simulink library "amg_clcd_lib"  (R2015b)
settings: Solver=ode3  SolverMode=SingleTasking  StartTime=0.0  StopTime=10.0  RelTol=1e-3
(part 1 of 3)
settings Model: Creator=Krisada  LastModifiedBy=Aimagin
settings DataIOCC: SaveFormat=Array  SignalLoggingSaveFormat=ModelDataLogs
settings OptimizationCC: ExpressionDepthLimit=2147483647  OptimizeModelRefInitCode=on  LifeSpan=1
settings DebuggingCC: UnderspecifiedInitializationDetection=Classic  MergeDetectMultiDrivingBlocksExec=none  SolverPrmCheckMsg=warning  FcnCallInpInsideContextMsg=UseLocalSettings  StateNameClashWarn=warning  StrictBusMsg=Warning
settings HardwareCC: ProdBitPerPointer=32  ProdLargestAtomicFloat=None  ProdIntDivRoundTo=Undefined  ProdWordSize=32  ProdHWDeviceType=ARM Compatible->Cortex - M4  TargetEndianess=LittleEndian  TargetHWDeviceType=ARM Compatible->Cortex - M4
settings RTWCC: SystemTargetFile=stm32f4.tlc  GenerateMakefile=off  TemplateMakefile=ert_default_tmf  Description=STM32F4 Target
settings CodeAppCC: IgnoreCustomStorageClasses=off  CustomSymbolStrType=$N$R$M  InternalIdentifier=Classic
settings STFCustomTargetCC: ModelReferenceCompliant=off  ConcurrentExecutionCompliant=off  GeneratePreprocessorConditionals=Use local settings  CombineOutputUpdateFcns=on  ERTCustomFileBanners=on  SupportContinuousTime=off  SupportNonInlinedSFcns=off  MATLABClassNameForMDSCustomization=Simulink.SoftwareTarget.ERTCustomization  CPPClassGenCompliant=off  GRTInterface=off  SystemTargetFile=stm32f4.tlc
settings ERTTargetCC: ModelReferenceCompliant=off  ParMdlRefBuildCompliant=off  CompOptLevelCompliant=off  ConcurrentExecutionCompliant=off  ERTFirstTimeCompliant=off  ModelStepFunctionPrototypeControlCompliant=off  CPPClassGenCompliant=off  UseToolchainInfoCompliant=off  ERTSrcFileBannerTemplate=stm32f4_code_template.cgt  ERTHdrFileBannerTemplate=stm32f4_code_template.cgt  ERTDataSrcFileTemplate=stm32f4_code_template.cgt  ERTDataHdrFileTemplate=stm32f4_code_template.cgt  ERTCustomFileTemplate=stm32f4_file_process.tlc
settings ConfigComp: CovModelRefEnable=Off

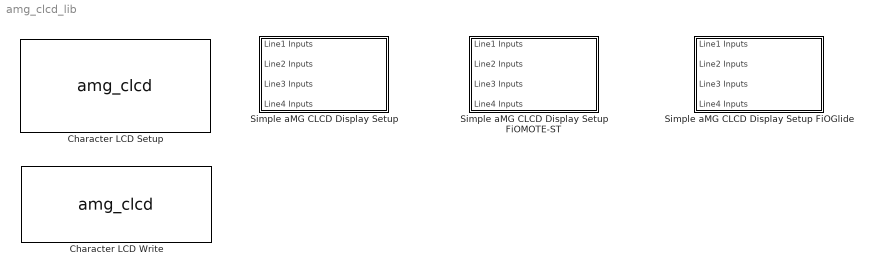
== system amg_clcd_lib ==
  Character LCD Setup : S-Function  FunctionName=amg_clcd  Parameters=module,configuration,inputtypearray,outputtypearray,confstr,sampletime,sampletimestr,blockid  SFunctionDeploymentMode=off  EnableBusSupport=off  mask(amg_clcd){configuration=Setup, module=1, model=amg CLCD Std, interface=4-bits, linecount=4, columncount=16, gpiotype=Push-pull, controlport=E, control_rs=7, control_rw=8, control_en=9, dataport_low=C, dataport=E, datalow0=8, datalow1=9, datalow2=10, datalow3=11, data0=12, data1=13, data2=14, data3=15, usestringbuffer=off, stringbuffer=<empty>, varname=, inputtypearray=[0], outputtypearray=[0], confstr=["4","4","16","PP","E","7","9","8","C","E","8","9","10","11","12","13","14","15","0","","0","0","1","0","1","0","0","0","0","stm32f0"], sampletime=-1, sampletimestr=0, blockid=CharacterLCDSetup}
      mask prompts: model "LCD model:"; linecount "Number of lines (2 or 4):"; columncount "Number of columns (16 or 20):"; gpiotype "GPIO Output type:"; controlport "GPIO control port:"; control_rs "GPIO control pin, RS:"; control_rw "GPIO control pin, RW:"; control_en "GPIO control pin, EN:"; dataport_low "GPIO data D[3:0] port"; dataport "GPIO data D[7:4] port"; datalow0 "GPIO data pin, D0:"; datalow1 "GPIO data pin, D1:"; datalow2 "GPIO data pin, D2:"; datalow3 "GPIO data pin, D3:"; data0 "GPIO data pin, D4:"; data1 "GPIO data pin, D5:"; data2 "GPIO data pin, D6:"; data3 "GPIO data pin, D7:"; usestringbuffer "Use string buffer"; stringbuffer "String buffer"; varname "Variable name"; inputtypearray "Input type array"; outputtypearray "Output type array"; confstr "Configuration string"; sampletime "Sample time (sec)"; sampletimestr "Compiled sample time (sec) in string"
      mask help:
      | Interface:
      |  - Select LCD data pin count to 4 or 8 line.
      |
      | Number of columns:
      |  - Select 16 for LCD 1x16, 2x16 or 4x16 characters.
      |  - Select 20 for LCD 1x20, 2x20 or 4x20 characters.
      |
      | GPIO Output type:
      |  - Select Push-Pull to drive 3.3V push-pull from MCU.
      |  - Select Open-Drain to allow external 5V pull-up.
      mask init:
      | amg_clcd_callback('init');
      mask Help: web(fullfile(waijungdocroot,'amg_clcd_setup.htm'), '-browser')
      mask TypeOptions configuration: Setup | Transaction
      mask Callback configuration: amg_clcd_callback('configuration');
      mask TypeOptions module: 1 | 2 | 3 | 4
      mask TypeOptions model: amg CLCD Std
      mask TypeOptions interface: 4-bits | 8-bits
      mask Callback interface: amg_clcd_callback('interface');
      mask TypeOptions gpiotype: Push-pull | Open-drain
      mask TypeOptions controlport: A | B | C | D | E | F | G | H | I
      mask TypeOptions control_rs: 0 | 1 | 2 | 3 | 4 | 5 | 6 | 7 | 8 | 9 | 10 | 11 | 12 | 13 | 14 | 15
      mask TypeOptions control_rw: 0 | 1 | 2 | 3 | 4 | 5 | 6 | 7 | 8 | 9 | 10 | 11 | 12 | 13 | 14 | 15
      mask TypeOptions control_en: 0 | 1 | 2 | 3 | 4 | 5 | 6 | 7 | 8 | 9 | 10 | 11 | 12 | 13 | 14 | 15
      mask TypeOptions dataport_low: A | B | C | D | E | F | G | H | I
      mask TypeOptions dataport: A | B | C | D | E | F | G | H | I
      mask TypeOptions datalow0: 0 | 1 | 2 | 3 | 4 | 5 | 6 | 7 | 8 | 9 | 10 | 11 | 12 | 13 | 14 | 15
      mask TypeOptions datalow1: 0 | 1 | 2 | 3 | 4 | 5 | 6 | 7 | 8 | 9 | 10 | 11 | 12 | 13 | 14 | 15
      mask TypeOptions datalow2: 0 | 1 | 2 | 3 | 4 | 5 | 6 | 7 | 8 | 9 | 10 | 11 | 12 | 13 | 14 | 15
      mask TypeOptions datalow3: 0 | 1 | 2 | 3 | 4 | 5 | 6 | 7 | 8 | 9 | 10 | 11 | 12 | 13 | 14 | 15
      mask TypeOptions data0: 0 | 1 | 2 | 3 | 4 | 5 | 6 | 7 | 8 | 9 | 10 | 11 | 12 | 13 | 14 | 15
      mask TypeOptions data1: 0 | 1 | 2 | 3 | 4 | 5 | 6 | 7 | 8 | 9 | 10 | 11 | 12 | 13 | 14 | 15
      mask TypeOptions data2: 0 | 1 | 2 | 3 | 4 | 5 | 6 | 7 | 8 | 9 | 10 | 11 | 12 | 13 | 14 | 15
      mask TypeOptions data3: 0 | 1 | 2 | 3 | 4 | 5 | 6 | 7 | 8 | 9 | 10 | 11 | 12 | 13 | 14 | 15
      mask Callback usestringbuffer: amg_clcd_callback('usestringbuffer');
      mask TypeOptions stringbuffer: <empty>
      mask Callback varname: amg_clcd_callback('varname');
      mask Callback confstr: amg_clcd_callback('confstr');
      mask Callback sampletime: amg_clcd_callback('sampletime');
      mask Callback sampletimestr: amg_clcd_callback('sampletimestr');
      mask Callback blockid: amg_clcd_callback('blockid');
      mask Display: text(0.5, 0.5, 'Module: CLCD1 (Setup)\nInterface: 4-bits\nCntrl: E7/E8/E9\nD[7:4]: E12/E13/E14/E15\nTs (sec): 0','ver','middle','hor','center');
  Character LCD Write : S-Function  FunctionName=amg_clcd  Parameters=module,configuration,inputtypearray,outputtypearray,confstr,sampletime,sampletimestr,blockid  SFunctionDeploymentMode=off  EnableBusSupport=off  mask(amg_clcd){configuration=Transaction, module=1, model=amg CLCD Std, interface=4-bits, linecount=4, columncount=20, gpiotype=Push-pull, controlport=E, control_rs=15, control_rw=13, control_en=11, dataport=A, data0=7, data1=5, data2=3, data3=1, usestringbuffer=off, stringbuffer=<empty>, varname=, inputtypearray=[4 -1 -1 -1 -1], outputtypearray=[0], confstr=["4","4","20","PP","E","15","11","13","","A","","","","","7","5","3","1","0","","1","0","0","0","1","0","0","0","0","stm32f0"], sampletime=-1, sampletimestr=0, blockid=CharacterLCDWrite}
      mask prompts: model "LCD model:"; linecount "Number of lines:"; columncount "Number of columns:"; gpiotype "GPIO Output type:"; controlport "GPIO control port:"; control_rs "GPIO control pin, RS:"; control_rw "GPIO control pin, RW:"; control_en "GPIO control pin, EN:"; dataport "GPIO data D[7:4] port"; data0 "GPIO data pin, D4:"; data1 "GPIO data pin, D5:"; data2 "GPIO data pin, D6:"; data3 "GPIO data pin, D7:"; usestringbuffer "Use string buffer"; stringbuffer "String buffer"; varname "Variable name"; inputtypearray "Input type array"; outputtypearray "Output type array"; confstr "Configuration string"; sampletime "Sample time (sec)"; sampletimestr "Compiled sample time (sec) in string"
      mask help:
      | Note for cmd:
      | 1 - Clear specified LCD line display before write data to LCD.
      | Otherwise (e.g. 0) - Write data without clearing LCD Line.
      |
      | Position:
      | x = 0, First Character (from left to right)
      | y = 0, Top Line
      mask init:
      | amg_clcd_callback('init');
      mask Help: web(fullfile(waijungdocroot,'amg_clcd_write.htm'), '-browser')
      mask TypeOptions configuration: Setup | Transaction
      mask Callback configuration: amg_clcd_callback('configuration');
      mask TypeOptions module: 1 | 2 | 3 | 4
      mask TypeOptions model: amg CLCD Std
      mask TypeOptions interface: 4-bits
      mask TypeOptions gpiotype: Push-pull | Open-drain
      mask TypeOptions controlport: A | B | C | D | E | F | G | H | I
      mask TypeOptions control_rs: 0 | 1 | 2 | 3 | 4 | 5 | 6 | 7 | 8 | 9 | 10 | 11 | 12 | 13 | 14 | 15
      mask TypeOptions control_rw: 0 | 1 | 2 | 3 | 4 | 5 | 6 | 7 | 8 | 9 | 10 | 11 | 12 | 13 | 14 | 15
      mask TypeOptions control_en: 0 | 1 | 2 | 3 | 4 | 5 | 6 | 7 | 8 | 9 | 10 | 11 | 12 | 13 | 14 | 15
      mask TypeOptions dataport: A | B | C | D | E | F | G | H | I
      mask TypeOptions data0: 0 | 1 | 2 | 3 | 4 | 5 | 6 | 7 | 8 | 9 | 10 | 11 | 12 | 13 | 14 | 15
      mask TypeOptions data1: 0 | 1 | 2 | 3 | 4 | 5 | 6 | 7 | 8 | 9 | 10 | 11 | 12 | 13 | 14 | 15
      mask TypeOptions data2: 0 | 1 | 2 | 3 | 4 | 5 | 6 | 7 | 8 | 9 | 10 | 11 | 12 | 13 | 14 | 15
      mask TypeOptions data3: 0 | 1 | 2 | 3 | 4 | 5 | 6 | 7 | 8 | 9 | 10 | 11 | 12 | 13 | 14 | 15
      mask Callback usestringbuffer: amg_clcd_callback('usestringbuffer');
      mask TypeOptions stringbuffer: Line1 | Line2 | Line3 | Line4 | Line1 | Line2 | Line3 | Line4 | Line1 | Line2 | Line3 | Line4 | <empty>
      mask Callback varname: amg_clcd_callback('varname');
      mask Callback confstr: amg_clcd_callback('confstr');
      mask Callback sampletime: amg_clcd_callback('sampletime');
      mask Callback sampletimestr: amg_clcd_callback('sampletimestr');
      mask Callback blockid: amg_clcd_callback('blockid');
      mask Display: text(0.5, 0.5, 'Module: CLCD1 (Write)\nTs (sec): 0','ver','middle','hor','center');port_label('input', 1,'cmd');port_label('input', 2,'xpos');port_label('input', 3,'ypos');port_label('input', 4,'str');
  Simple aMG CLCD Display Setup : Subsystem
      settings: CopyFcn=set_param(gcbh, 'LinkStatus', 'none')
  Simple aMG CLCD Display Setup FiOGlide : Subsystem
      settings: CopyFcn=set_param(gcbh, 'LinkStatus', 'none')
  Simple aMG CLCD Display Setup FiOMOTE-ST : Subsystem
      settings: CopyFcn=set_param(gcbh, 'LinkStatus', 'none')

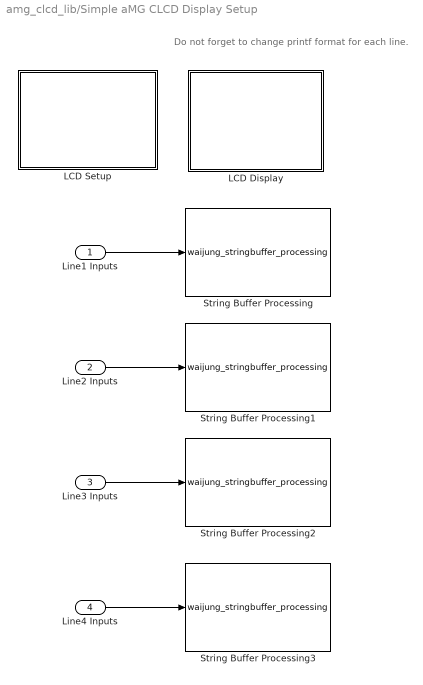
== system amg_clcd_lib/Simple aMG CLCD Display Setup ==
  note: Do not forget to change printf format for each line.
  Line1 Inputs : Inport
  Line2 Inputs : Inport  Port=2
  Line3 Inputs : Inport  Port=3
  Line4 Inputs : Inport  Port=4
  LCD Display : Subsystem
  LCD Setup : Subsystem
  String Buffer Processing : S-Function  FunctionName=waijung_stringbuffer_processing  Parameters=configuration,varname,sformat,porttypes,portcount,inputtypearray,outputtypearray,sampletime,sampletimestr,blockid  SFunctionDeploymentMode=off  EnableBusSupport=off  mask(waijung_stringbuffer_processing){configuration=sprintf, storagename=Line1, sformat='%u', enableoutput=off, varname=SimpleaMGCLCDDisplaySetupLCDSetupVolatileDataStorage_Line1, inputtypearray=[1 -1], outputtypearray=[0], porttypes=["uint32_t"], portcount=1, sampletime=-1, sampletimestr=0, blockid=SimpleaMGCLCDDisplaySetupStringBufferProcessing}
      mask prompts: configuration "Function"; storagename "String buffer"; sformat "Printf format"; enableoutput "Enable output status"; varname "Variable name"; inputtypearray "Input type array"; outputtypearray "Output type array"; porttypes "Port type list"; portcount "Port type count"; sampletime "Sample time (sec)"; sampletimestr "Compiled sample time (sec) in string"
      mask help:
      | This block implements string processing, sprintf/ sscanf command.
      | Supported format:
      | %u, %i, %o, %x: uint32
      | %d: int32
      | %e, %g, %f: single
      | %c: int8
      |
      | Status:
      |  0: Failed.
      |  Non-zero: Success.
      mask init:
      | waijung_stringbuffer_processing_callback('init');
      mask Help: web(fullfile(waijungdocroot,'String_Buffer_Processing.htm'))
      mask TypeOptions configuration: sprintf | sscanf
      mask Callback configuration: waijung_stringbuffer_processing_callback('configuration');
      mask TypeOptions storagename: Line1 | Line2 | Line3 | Line4 | Line1 | Line2 | Line3 | Line4 | Line1 | Line2 | Line3 | Line4 | <output>
      mask Callback sformat: waijung_stringbuffer_processing_callback('sformat');
      mask Callback enableoutput: waijung_stringbuffer_processing_callback('enableoutput');
      mask Callback sampletime: waijung_stringbuffer_processing_callback('sampletime');
      mask Callback sampletimestr: waijung_stringbuffer_processing_callback('sampletimestr');
      mask Callback blockid: waijung_stringbuffer_processing_callback('blockid');
      mask Display: text(0.5, 0.5, '[ sprintf ]\nBuffer: Line1\nTs (sec): 0','ver','middle','hor','center');port_label('input', 1,'%u');
  String Buffer Processing1 : S-Function  FunctionName=waijung_stringbuffer_processing  Parameters=configuration,varname,sformat,porttypes,portcount,inputtypearray,outputtypearray,sampletime,sampletimestr,blockid  SFunctionDeploymentMode=off  EnableBusSupport=off  mask(waijung_stringbuffer_processing){configuration=sprintf, storagename=Line2, sformat='%u', enableoutput=off, varname=SimpleaMGCLCDDisplaySetupLCDSetupVolatileDataStorage1_Line2, inputtypearray=[1 -1], outputtypearray=[0], porttypes=["uint32_t"], portcount=1, sampletime=-1, sampletimestr=0, blockid=SimpleaMGCLCDDisplaySetupStringBufferProcessing1}
      mask prompts: configuration "Function"; storagename "String buffer"; sformat "Printf format"; enableoutput "Enable output status"; varname "Variable name"; inputtypearray "Input type array"; outputtypearray "Output type array"; porttypes "Port type list"; portcount "Port type count"; sampletime "Sample time (sec)"; sampletimestr "Compiled sample time (sec) in string"
      mask help:
      | This block implements string processing, sprintf/ sscanf command.
      | Supported format:
      | %u, %i, %o, %x: uint32
      | %d: int32
      | %e, %g, %f: single
      | %c: int8
      |
      | Status:
      |  0: Failed.
      |  Non-zero: Success.
      mask init:
      | waijung_stringbuffer_processing_callback('init');
      mask Help: web(fullfile(waijungdocroot,'String_Buffer_Processing.htm'))
      mask TypeOptions configuration: sprintf | sscanf
      mask Callback configuration: waijung_stringbuffer_processing_callback('configuration');
      mask TypeOptions storagename: Line1 | Line2 | Line3 | Line4 | Line1 | Line2 | Line3 | Line4 | Line1 | Line2 | Line3 | Line4 | <output>
      mask Callback sformat: waijung_stringbuffer_processing_callback('sformat');
      mask Callback enableoutput: waijung_stringbuffer_processing_callback('enableoutput');
      mask Callback sampletime: waijung_stringbuffer_processing_callback('sampletime');
      mask Callback sampletimestr: waijung_stringbuffer_processing_callback('sampletimestr');
      mask Callback blockid: waijung_stringbuffer_processing_callback('blockid');
      mask Display: text(0.5, 0.5, '[ sprintf ]\nBuffer: Line2\nTs (sec): 0','ver','middle','hor','center');port_label('input', 1,'%u');
  String Buffer Processing2 : S-Function  FunctionName=waijung_stringbuffer_processing  Parameters=configuration,varname,sformat,porttypes,portcount,inputtypearray,outputtypearray,sampletime,sampletimestr,blockid  SFunctionDeploymentMode=off  EnableBusSupport=off  mask(waijung_stringbuffer_processing){configuration=sprintf, storagename=Line3, sformat='%u', enableoutput=off, varname=SimpleaMGCLCDDisplaySetupLCDSetupVolatileDataStorage2_Line3, inputtypearray=[1 -1], outputtypearray=[0], porttypes=["uint32_t"], portcount=1, sampletime=-1, sampletimestr=0, blockid=SimpleaMGCLCDDisplaySetupStringBufferProcessing2}
      mask prompts: configuration "Function"; storagename "String buffer"; sformat "Printf format"; enableoutput "Enable output status"; varname "Variable name"; inputtypearray "Input type array"; outputtypearray "Output type array"; porttypes "Port type list"; portcount "Port type count"; sampletime "Sample time (sec)"; sampletimestr "Compiled sample time (sec) in string"
      mask help:
      | This block implements string processing, sprintf/ sscanf command.
      | Supported format:
      | %u, %i, %o, %x: uint32
      | %d: int32
      | %e, %g, %f: single
      | %c: int8
      |
      | Status:
      |  0: Failed.
      |  Non-zero: Success.
      mask init:
      | waijung_stringbuffer_processing_callback('init');
      mask Help: web(fullfile(waijungdocroot,'String_Buffer_Processing.htm'))
      mask TypeOptions configuration: sprintf | sscanf
      mask Callback configuration: waijung_stringbuffer_processing_callback('configuration');
      mask TypeOptions storagename: Line1 | Line2 | Line3 | Line4 | Line1 | Line2 | Line3 | Line4 | Line1 | Line2 | Line3 | Line4 | <output>
      mask Callback sformat: waijung_stringbuffer_processing_callback('sformat');
      mask Callback enableoutput: waijung_stringbuffer_processing_callback('enableoutput');
      mask Callback sampletime: waijung_stringbuffer_processing_callback('sampletime');
      mask Callback sampletimestr: waijung_stringbuffer_processing_callback('sampletimestr');
      mask Callback blockid: waijung_stringbuffer_processing_callback('blockid');
      mask Display: text(0.5, 0.5, '[ sprintf ]\nBuffer: Line3\nTs (sec): 0','ver','middle','hor','center');port_label('input', 1,'%u');
  String Buffer Processing3 : S-Function  FunctionName=waijung_stringbuffer_processing  Parameters=configuration,varname,sformat,porttypes,portcount,inputtypearray,outputtypearray,sampletime,sampletimestr,blockid  SFunctionDeploymentMode=off  EnableBusSupport=off  mask(waijung_stringbuffer_processing){configuration=sprintf, storagename=Line4, sformat='%u', enableoutput=off, varname=SimpleaMGCLCDDisplaySetupLCDSetupVolatileDataStorage3_Line4, inputtypearray=[1 -1], outputtypearray=[0], porttypes=["uint32_t"], portcount=1, sampletime=-1, sampletimestr=0, blockid=SimpleaMGCLCDDisplaySetupStringBufferProcessing3}
      mask prompts: configuration "Function"; storagename "String buffer"; sformat "Printf format"; enableoutput "Enable output status"; varname "Variable name"; inputtypearray "Input type array"; outputtypearray "Output type array"; porttypes "Port type list"; portcount "Port type count"; sampletime "Sample time (sec)"; sampletimestr "Compiled sample time (sec) in string"
      mask help:
      | This block implements string processing, sprintf/ sscanf command.
      | Supported format:
      | %u, %i, %o, %x: uint32
      | %d: int32
      | %e, %g, %f: single
      | %c: int8
      |
      | Status:
      |  0: Failed.
      |  Non-zero: Success.
      mask init:
      | waijung_stringbuffer_processing_callback('init');
      mask Help: web(fullfile(waijungdocroot,'String_Buffer_Processing.htm'))
      mask TypeOptions configuration: sprintf | sscanf
      mask Callback configuration: waijung_stringbuffer_processing_callback('configuration');
      mask TypeOptions storagename: Line1 | Line2 | Line3 | Line4 | Line1 | Line2 | Line3 | Line4 | Line1 | Line2 | Line3 | Line4 | <output>
      mask Callback sformat: waijung_stringbuffer_processing_callback('sformat');
      mask Callback enableoutput: waijung_stringbuffer_processing_callback('enableoutput');
      mask Callback sampletime: waijung_stringbuffer_processing_callback('sampletime');
      mask Callback sampletimestr: waijung_stringbuffer_processing_callback('sampletimestr');
      mask Callback blockid: waijung_stringbuffer_processing_callback('blockid');
      mask Display: text(0.5, 0.5, '[ sprintf ]\nBuffer: Line4\nTs (sec): 0','ver','middle','hor','center');port_label('input', 1,'%u');
  wires:
  Line1 Inputs/1 -> String Buffer Processing/1
  Line2 Inputs/1 -> String Buffer Processing1/1
  Line3 Inputs/1 -> String Buffer Processing2/1
  Line4 Inputs/1 -> String Buffer Processing3/1

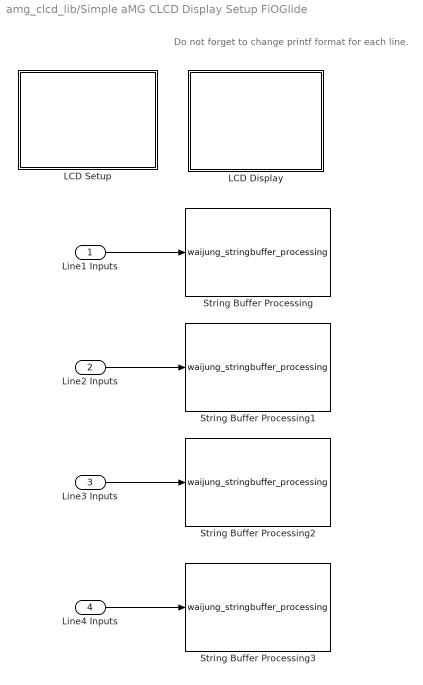
== system amg_clcd_lib/Simple aMG CLCD Display Setup FiOGlide ==
  note: Do not forget to change printf format for each line.
  Line1 Inputs : Inport
  Line2 Inputs : Inport  Port=2
  Line3 Inputs : Inport  Port=3
  Line4 Inputs : Inport  Port=4
  LCD Display : Subsystem
  LCD Setup : Subsystem
  String Buffer Processing : S-Function  FunctionName=waijung_stringbuffer_processing  Parameters=configuration,varname,sformat,porttypes,portcount,inputtypearray,outputtypearray,sampletime,sampletimestr,blockid  SFunctionDeploymentMode=off  EnableBusSupport=off  mask(waijung_stringbuffer_processing){configuration=sprintf, storagename=Line1, sformat='%u', enableoutput=off, varname=SimpleaMGCLCDDisplaySetupLCDSetupVolatileDataStorage_Line1, inputtypearray=[1 -1], outputtypearray=[0], porttypes=["uint32_t"], portcount=1, sampletime=-1, sampletimestr=0, blockid=SimpleaMGCLCDDisplaySetupStringBufferProcessing}
      mask prompts: configuration "Function"; storagename "String buffer"; sformat "Printf format"; enableoutput "Enable output status"; varname "Variable name"; inputtypearray "Input type array"; outputtypearray "Output type array"; porttypes "Port type list"; portcount "Port type count"; sampletime "Sample time (sec)"; sampletimestr "Compiled sample time (sec) in string"
      mask help:
      | This block implements string processing, sprintf/ sscanf command.
      | Supported format:
      | %u, %i, %o, %x: uint32
      | %d: int32
      | %e, %g, %f: single
      | %c: int8
      |
      | Status:
      |  0: Failed.
      |  Non-zero: Success.
      mask init:
      | waijung_stringbuffer_processing_callback('init');
      mask Help: web(fullfile(waijungdocroot,'String_Buffer_Processing.htm'))
      mask TypeOptions configuration: sprintf | sscanf
      mask Callback configuration: waijung_stringbuffer_processing_callback('configuration');
      mask TypeOptions storagename: Line1 | Line2 | Line3 | Line4 | Line1 | Line2 | Line3 | Line4 | Line1 | Line2 | Line3 | Line4 | <output>
      mask Callback sformat: waijung_stringbuffer_processing_callback('sformat');
      mask Callback enableoutput: waijung_stringbuffer_processing_callback('enableoutput');
      mask Callback sampletime: waijung_stringbuffer_processing_callback('sampletime');
      mask Callback sampletimestr: waijung_stringbuffer_processing_callback('sampletimestr');
      mask Callback blockid: waijung_stringbuffer_processing_callback('blockid');
      mask Display: text(0.5, 0.5, '[ sprintf ]\nBuffer: Line1\nTs (sec): 0','ver','middle','hor','center');port_label('input', 1,'%u');
  String Buffer Processing1 : S-Function  FunctionName=waijung_stringbuffer_processing  Parameters=configuration,varname,sformat,porttypes,portcount,inputtypearray,outputtypearray,sampletime,sampletimestr,blockid  SFunctionDeploymentMode=off  EnableBusSupport=off  mask(waijung_stringbuffer_processing){configuration=sprintf, storagename=Line2, sformat='%u', enableoutput=off, varname=SimpleaMGCLCDDisplaySetupLCDSetupVolatileDataStorage1_Line2, inputtypearray=[1 -1], outputtypearray=[0], porttypes=["uint32_t"], portcount=1, sampletime=-1, sampletimestr=0, blockid=SimpleaMGCLCDDisplaySetupStringBufferProcessing1}
      mask prompts: configuration "Function"; storagename "String buffer"; sformat "Printf format"; enableoutput "Enable output status"; varname "Variable name"; inputtypearray "Input type array"; outputtypearray "Output type array"; porttypes "Port type list"; portcount "Port type count"; sampletime "Sample time (sec)"; sampletimestr "Compiled sample time (sec) in string"
      mask help:
      | This block implements string processing, sprintf/ sscanf command.
      | Supported format:
      | %u, %i, %o, %x: uint32
      | %d: int32
      | %e, %g, %f: single
      | %c: int8
      |
      | Status:
      |  0: Failed.
      |  Non-zero: Success.
      mask init:
      | waijung_stringbuffer_processing_callback('init');
      mask Help: web(fullfile(waijungdocroot,'String_Buffer_Processing.htm'))
      mask TypeOptions configuration: sprintf | sscanf
      mask Callback configuration: waijung_stringbuffer_processing_callback('configuration');
      mask TypeOptions storagename: Line1 | Line2 | Line3 | Line4 | Line1 | Line2 | Line3 | Line4 | Line1 | Line2 | Line3 | Line4 | <output>
      mask Callback sformat: waijung_stringbuffer_processing_callback('sformat');
      mask Callback enableoutput: waijung_stringbuffer_processing_callback('enableoutput');
      mask Callback sampletime: waijung_stringbuffer_processing_callback('sampletime');
      mask Callback sampletimestr: waijung_stringbuffer_processing_callback('sampletimestr');
      mask Callback blockid: waijung_stringbuffer_processing_callback('blockid');
      mask Display: text(0.5, 0.5, '[ sprintf ]\nBuffer: Line2\nTs (sec): 0','ver','middle','hor','center');port_label('input', 1,'%u');
  String Buffer Processing2 : S-Function  FunctionName=waijung_stringbuffer_processing  Parameters=configuration,varname,sformat,porttypes,portcount,inputtypearray,outputtypearray,sampletime,sampletimestr,blockid  SFunctionDeploymentMode=off  EnableBusSupport=off  mask(waijung_stringbuffer_processing){configuration=sprintf, storagename=Line3, sformat='%u', enableoutput=off, varname=SimpleaMGCLCDDisplaySetupLCDSetupVolatileDataStorage2_Line3, inputtypearray=[1 -1], outputtypearray=[0], porttypes=["uint32_t"], portcount=1, sampletime=-1, sampletimestr=0, blockid=SimpleaMGCLCDDisplaySetupStringBufferProcessing2}
      mask prompts: configuration "Function"; storagename "String buffer"; sformat "Printf format"; enableoutput "Enable output status"; varname "Variable name"; inputtypearray "Input type array"; outputtypearray "Output type array"; porttypes "Port type list"; portcount "Port type count"; sampletime "Sample time (sec)"; sampletimestr "Compiled sample time (sec) in string"
      mask help:
      | This block implements string processing, sprintf/ sscanf command.
      | Supported format:
      | %u, %i, %o, %x: uint32
      | %d: int32
      | %e, %g, %f: single
      | %c: int8
      |
      | Status:
      |  0: Failed.
      |  Non-zero: Success.
      mask init:
      | waijung_stringbuffer_processing_callback('init');
      mask Help: web(fullfile(waijungdocroot,'String_Buffer_Processing.htm'))
      mask TypeOptions configuration: sprintf | sscanf
      mask Callback configuration: waijung_stringbuffer_processing_callback('configuration');
      mask TypeOptions storagename: Line1 | Line2 | Line3 | Line4 | Line1 | Line2 | Line3 | Line4 | Line1 | Line2 | Line3 | Line4 | <output>
      mask Callback sformat: waijung_stringbuffer_processing_callback('sformat');
      mask Callback enableoutput: waijung_stringbuffer_processing_callback('enableoutput');
      mask Callback sampletime: waijung_stringbuffer_processing_callback('sampletime');
      mask Callback sampletimestr: waijung_stringbuffer_processing_callback('sampletimestr');
      mask Callback blockid: waijung_stringbuffer_processing_callback('blockid');
      mask Display: text(0.5, 0.5, '[ sprintf ]\nBuffer: Line3\nTs (sec): 0','ver','middle','hor','center');port_label('input', 1,'%u');
  String Buffer Processing3 : S-Function  FunctionName=waijung_stringbuffer_processing  Parameters=configuration,varname,sformat,porttypes,portcount,inputtypearray,outputtypearray,sampletime,sampletimestr,blockid  SFunctionDeploymentMode=off  EnableBusSupport=off  mask(waijung_stringbuffer_processing){configuration=sprintf, storagename=Line4, sformat='%u', enableoutput=off, varname=SimpleaMGCLCDDisplaySetupLCDSetupVolatileDataStorage3_Line4, inputtypearray=[1 -1], outputtypearray=[0], porttypes=["uint32_t"], portcount=1, sampletime=-1, sampletimestr=0, blockid=SimpleaMGCLCDDisplaySetupStringBufferProcessing3}
      mask prompts: configuration "Function"; storagename "String buffer"; sformat "Printf format"; enableoutput "Enable output status"; varname "Variable name"; inputtypearray "Input type array"; outputtypearray "Output type array"; porttypes "Port type list"; portcount "Port type count"; sampletime "Sample time (sec)"; sampletimestr "Compiled sample time (sec) in string"
      mask help:
      | This block implements string processing, sprintf/ sscanf command.
      | Supported format:
      | %u, %i, %o, %x: uint32
      | %d: int32
      | %e, %g, %f: single
      | %c: int8
      |
      | Status:
      |  0: Failed.
      |  Non-zero: Success.
      mask init:
      | waijung_stringbuffer_processing_callback('init');
      mask Help: web(fullfile(waijungdocroot,'String_Buffer_Processing.htm'))
      mask TypeOptions configuration: sprintf | sscanf
      mask Callback configuration: waijung_stringbuffer_processing_callback('configuration');
      mask TypeOptions storagename: Line1 | Line2 | Line3 | Line4 | Line1 | Line2 | Line3 | Line4 | Line1 | Line2 | Line3 | Line4 | <output>
      mask Callback sformat: waijung_stringbuffer_processing_callback('sformat');
      mask Callback enableoutput: waijung_stringbuffer_processing_callback('enableoutput');
      mask Callback sampletime: waijung_stringbuffer_processing_callback('sampletime');
      mask Callback sampletimestr: waijung_stringbuffer_processing_callback('sampletimestr');
      mask Callback blockid: waijung_stringbuffer_processing_callback('blockid');
      mask Display: text(0.5, 0.5, '[ sprintf ]\nBuffer: Line4\nTs (sec): 0','ver','middle','hor','center');port_label('input', 1,'%u');
  wires:
  Line4 Inputs/1 -> String Buffer Processing3/1
  Line3 Inputs/1 -> String Buffer Processing2/1
  Line2 Inputs/1 -> String Buffer Processing1/1
  Line1 Inputs/1 -> String Buffer Processing/1

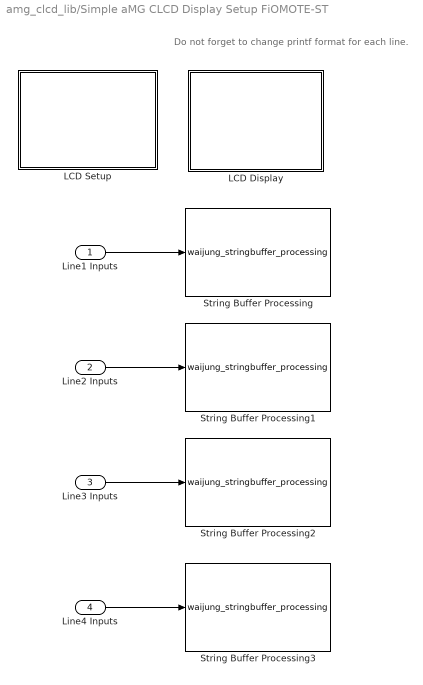
== system amg_clcd_lib/Simple aMG CLCD Display Setup FiOMOTE-ST ==
  note: Do not forget to change printf format for each line.
  Line1 Inputs : Inport
  Line2 Inputs : Inport  Port=2
  Line3 Inputs : Inport  Port=3
  Line4 Inputs : Inport  Port=4
  LCD Display : Subsystem
  LCD Setup : Subsystem
  String Buffer Processing : S-Function  FunctionName=waijung_stringbuffer_processing  Parameters=configuration,varname,sformat,porttypes,portcount,inputtypearray,outputtypearray,sampletime,sampletimestr,blockid  SFunctionDeploymentMode=off  EnableBusSupport=off  mask(waijung_stringbuffer_processing){configuration=sprintf, storagename=Line1, sformat='%u', enableoutput=off, varname=SimpleaMGCLCDDisplaySetupLCDSetupVolatileDataStorage_Line1, inputtypearray=[1 -1], outputtypearray=[0], porttypes=["uint32_t"], portcount=1, sampletime=-1, sampletimestr=0, blockid=SimpleaMGCLCDDisplaySetupStringBufferProcessing}
      mask prompts: configuration "Function"; storagename "String buffer"; sformat "Printf format"; enableoutput "Enable output status"; varname "Variable name"; inputtypearray "Input type array"; outputtypearray "Output type array"; porttypes "Port type list"; portcount "Port type count"; sampletime "Sample time (sec)"; sampletimestr "Compiled sample time (sec) in string"
      mask help:
      | This block implements string processing, sprintf/ sscanf command.
      | Supported format:
      | %u, %i, %o, %x: uint32
      | %d: int32
      | %e, %g, %f: single
      | %c: int8
      |
      | Status:
      |  0: Failed.
      |  Non-zero: Success.
      mask init:
      | waijung_stringbuffer_processing_callback('init');
      mask Help: web(fullfile(waijungdocroot,'String_Buffer_Processing.htm'))
      mask TypeOptions configuration: sprintf | sscanf
      mask Callback configuration: waijung_stringbuffer_processing_callback('configuration');
      mask TypeOptions storagename: Line1 | Line2 | Line3 | Line4 | Line1 | Line2 | Line3 | Line4 | <output>
      mask Callback sformat: waijung_stringbuffer_processing_callback('sformat');
      mask Callback enableoutput: waijung_stringbuffer_processing_callback('enableoutput');
      mask Callback sampletime: waijung_stringbuffer_processing_callback('sampletime');
      mask Callback sampletimestr: waijung_stringbuffer_processing_callback('sampletimestr');
      mask Callback blockid: waijung_stringbuffer_processing_callback('blockid');
      mask Display: text(0.5, 0.5, '[ sprintf ]\nBuffer: Line1\nTs (sec): 0','ver','middle','hor','center');port_label('input', 1,'%u');
  String Buffer Processing1 : S-Function  FunctionName=waijung_stringbuffer_processing  Parameters=configuration,varname,sformat,porttypes,portcount,inputtypearray,outputtypearray,sampletime,sampletimestr,blockid  SFunctionDeploymentMode=off  EnableBusSupport=off  mask(waijung_stringbuffer_processing){configuration=sprintf, storagename=Line2, sformat='%u', enableoutput=off, varname=SimpleaMGCLCDDisplaySetupLCDSetupVolatileDataStorage1_Line2, inputtypearray=[1 -1], outputtypearray=[0], porttypes=["uint32_t"], portcount=1, sampletime=-1, sampletimestr=0, blockid=SimpleaMGCLCDDisplaySetupStringBufferProcessing1}
      mask prompts: configuration "Function"; storagename "String buffer"; sformat "Printf format"; enableoutput "Enable output status"; varname "Variable name"; inputtypearray "Input type array"; outputtypearray "Output type array"; porttypes "Port type list"; portcount "Port type count"; sampletime "Sample time (sec)"; sampletimestr "Compiled sample time (sec) in string"
      mask help:
      | This block implements string processing, sprintf/ sscanf command.
      | Supported format:
      | %u, %i, %o, %x: uint32
      | %d: int32
      | %e, %g, %f: single
      | %c: int8
      |
      | Status:
      |  0: Failed.
      |  Non-zero: Success.
      mask init:
      | waijung_stringbuffer_processing_callback('init');
      mask Help: web(fullfile(waijungdocroot,'String_Buffer_Processing.htm'))
      mask TypeOptions configuration: sprintf | sscanf
      mask Callback configuration: waijung_stringbuffer_processing_callback('configuration');
      mask TypeOptions storagename: Line1 | Line2 | Line3 | Line4 | Line1 | Line2 | Line3 | Line4 | <output>
      mask Callback sformat: waijung_stringbuffer_processing_callback('sformat');
      mask Callback enableoutput: waijung_stringbuffer_processing_callback('enableoutput');
      mask Callback sampletime: waijung_stringbuffer_processing_callback('sampletime');
      mask Callback sampletimestr: waijung_stringbuffer_processing_callback('sampletimestr');
      mask Callback blockid: waijung_stringbuffer_processing_callback('blockid');
      mask Display: text(0.5, 0.5, '[ sprintf ]\nBuffer: Line2\nTs (sec): 0','ver','middle','hor','center');port_label('input', 1,'%u');
  String Buffer Processing2 : S-Function  FunctionName=waijung_stringbuffer_processing  Parameters=configuration,varname,sformat,porttypes,portcount,inputtypearray,outputtypearray,sampletime,sampletimestr,blockid  SFunctionDeploymentMode=off  EnableBusSupport=off  mask(waijung_stringbuffer_processing){configuration=sprintf, storagename=Line3, sformat='%u', enableoutput=off, varname=SimpleaMGCLCDDisplaySetupLCDSetupVolatileDataStorage2_Line3, inputtypearray=[1 -1], outputtypearray=[0], porttypes=["uint32_t"], portcount=1, sampletime=-1, sampletimestr=0, blockid=SimpleaMGCLCDDisplaySetupStringBufferProcessing2}
      mask prompts: configuration "Function"; storagename "String buffer"; sformat "Printf format"; enableoutput "Enable output status"; varname "Variable name"; inputtypearray "Input type array"; outputtypearray "Output type array"; porttypes "Port type list"; portcount "Port type count"; sampletime "Sample time (sec)"; sampletimestr "Compiled sample time (sec) in string"
      mask help:
      | This block implements string processing, sprintf/ sscanf command.
      | Supported format:
      | %u, %i, %o, %x: uint32
      | %d: int32
      | %e, %g, %f: single
      | %c: int8
      |
      | Status:
      |  0: Failed.
      |  Non-zero: Success.
      mask init:
      | waijung_stringbuffer_processing_callback('init');
      mask Help: web(fullfile(waijungdocroot,'String_Buffer_Processing.htm'))
      mask TypeOptions configuration: sprintf | sscanf
      mask Callback configuration: waijung_stringbuffer_processing_callback('configuration');
      mask TypeOptions storagename: Line1 | Line2 | Line3 | Line4 | Line1 | Line2 | Line3 | Line4 | <output>
      mask Callback sformat: waijung_stringbuffer_processing_callback('sformat');
      mask Callback enableoutput: waijung_stringbuffer_processing_callback('enableoutput');
      mask Callback sampletime: waijung_stringbuffer_processing_callback('sampletime');
      mask Callback sampletimestr: waijung_stringbuffer_processing_callback('sampletimestr');
      mask Callback blockid: waijung_stringbuffer_processing_callback('blockid');
      mask Display: text(0.5, 0.5, '[ sprintf ]\nBuffer: Line3\nTs (sec): 0','ver','middle','hor','center');port_label('input', 1,'%u');
  String Buffer Processing3 : S-Function  FunctionName=waijung_stringbuffer_processing  Parameters=configuration,varname,sformat,porttypes,portcount,inputtypearray,outputtypearray,sampletime,sampletimestr,blockid  SFunctionDeploymentMode=off  EnableBusSupport=off  mask(waijung_stringbuffer_processing){configuration=sprintf, storagename=Line4, sformat='%u', enableoutput=off, varname=SimpleaMGCLCDDisplaySetupLCDSetupVolatileDataStorage3_Line4, inputtypearray=[1 -1], outputtypearray=[0], porttypes=["uint32_t"], portcount=1, sampletime=-1, sampletimestr=0, blockid=SimpleaMGCLCDDisplaySetupStringBufferProcessing3}
      mask prompts: configuration "Function"; storagename "String buffer"; sformat "Printf format"; enableoutput "Enable output status"; varname "Variable name"; inputtypearray "Input type array"; outputtypearray "Output type array"; porttypes "Port type list"; portcount "Port type count"; sampletime "Sample time (sec)"; sampletimestr "Compiled sample time (sec) in string"
      mask help:
      | This block implements string processing, sprintf/ sscanf command.
      | Supported format:
      | %u, %i, %o, %x: uint32
      | %d: int32
      | %e, %g, %f: single
      | %c: int8
      |
      | Status:
      |  0: Failed.
      |  Non-zero: Success.
      mask init:
      | waijung_stringbuffer_processing_callback('init');
      mask Help: web(fullfile(waijungdocroot,'String_Buffer_Processing.htm'))
      mask TypeOptions configuration: sprintf | sscanf
      mask Callback configuration: waijung_stringbuffer_processing_callback('configuration');
      mask TypeOptions storagename: Line1 | Line2 | Line3 | Line4 | Line1 | Line2 | Line3 | Line4 | <output>
      mask Callback sformat: waijung_stringbuffer_processing_callback('sformat');
      mask Callback enableoutput: waijung_stringbuffer_processing_callback('enableoutput');
      mask Callback sampletime: waijung_stringbuffer_processing_callback('sampletime');
      mask Callback sampletimestr: waijung_stringbuffer_processing_callback('sampletimestr');
      mask Callback blockid: waijung_stringbuffer_processing_callback('blockid');
      mask Display: text(0.5, 0.5, '[ sprintf ]\nBuffer: Line4\nTs (sec): 0','ver','middle','hor','center');port_label('input', 1,'%u');
  wires:
  Line4 Inputs/1 -> String Buffer Processing3/1
  Line3 Inputs/1 -> String Buffer Processing2/1
  Line2 Inputs/1 -> String Buffer Processing1/1
  Line1 Inputs/1 -> String Buffer Processing/1
